simulink model "test_libMdl_TrainEndDataGenerator"  (R2018a)
settings: Solver=FixedStepDiscrete  StartTime=0  StopTime=t_end  FixedStep=0.1  RelTol=1e-3
PreLoadFcn:
  | init_test_libMdl_TrainEndDataGenerator
InitFcn:
  | init_test_libMdl_TrainEndDataGenerator
values from neighbouring files (symbols this model uses):
  a_train_front = [0;0;0]    [init_test_libMdl_TrainEndDataGenerator.m]
  front_track_id = 1    [init_test_libMdl_TrainEndDataGenerator.m]
  v_train_front = 36    [init_test_libMdl_TrainEndDataGenerator.m]
libraries: simulink x1, libMdl_TrainEndDataGenerator x1
settings Model: SimulationMode=accelerator  PauseTimes=224  Creator=hwinter  LastModifiedBy=Hanno
settings DataIOCC: SaveOutput=off  SignalLogging=off  DSMLogging=off  SaveTime=off
settings DebuggingCC: ReadBeforeWriteMsg=DisableAll  WriteAfterWriteMsg=DisableAll  WriteAfterReadMsg=DisableAll  MultiTaskDSMMsg=none
settings HardwareCC: ProdBitPerLong=64  ProdHWDeviceType=Intel->x86-64 (Linux 64)  TargetBitPerPointer=64  TargetBitPerSizeT=64  TargetBitPerPtrDiffT=64  TargetLongLongMode=on  TargetIntDivRoundTo=Zero  TargetEndianess=LittleEndian  TargetWordSize=64  TargetHWDeviceType=MATLAB Host  ProdEqTarget=off
settings SFSimCC: SFSimEcho=off
settings RTWCC: SystemTargetFile=rsim.tlc  TemplateMakefile=rsim_default_tmf  Description=Rapid Simulation Target
settings CodeAppCC: StateflowObjectComments=on
settings RSimTargetCC: TargetLangStandard=C99 (ISO)  GeneratePreprocessorConditionals=Use local settings

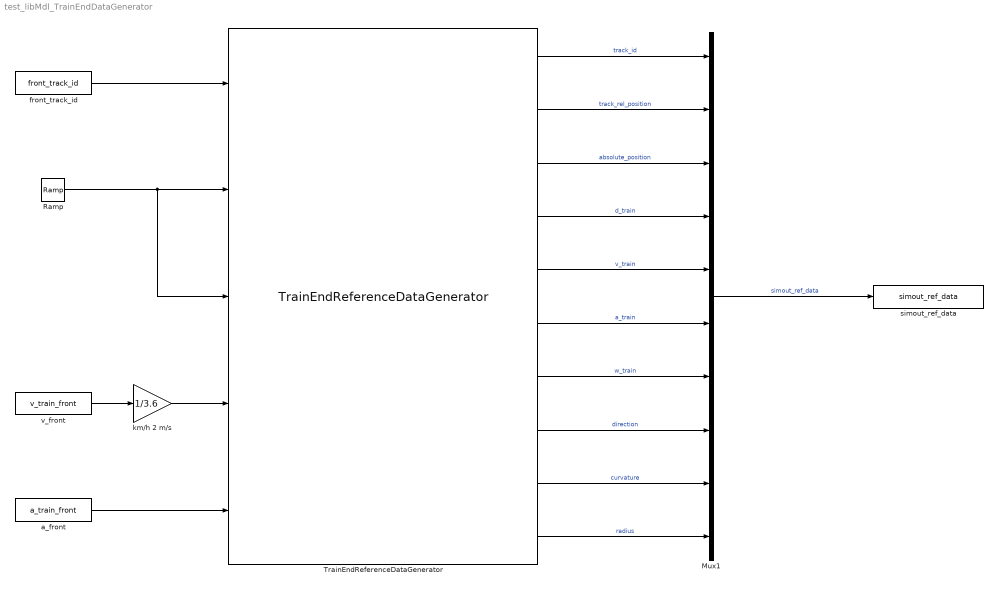
== system test_libMdl_TrainEndDataGenerator ==
  Mux1 : Mux  Inputs=10
  Ramp : simulink/Sources/Ramp  slope=v_train_front/3.6  start=0  InitialOutput=0
  TrainEndReferenceDataGenerator : libMdl_TrainEndDataGenerator/TrainEndReferenceDataGenerator  mv_train_length=train_length  mv_track_map=mat_track_map  mv_track_map_rot_angle=phi_track
  a_front : Constant  Value=a_train_front
  front_track_id : Constant  Value=front_track_id
  km/h 2 m/s : Gain  Gain=1/3.6
  simout_ref_data : ToWorkspace  VariableName=simout_ref_data  SaveFormat=Timeseries  SampleTime=-1
  v_front : Constant  Value=v_train_front
  wires:
  v_front/1 -> km/h 2 m/s/1
  TrainEndReferenceDataGenerator/6 -> Mux1/6  "a_train"
  TrainEndReferenceDataGenerator/7 -> Mux1/7  "w_train"
  TrainEndReferenceDataGenerator/3 -> Mux1/3  "absolute_position"
  TrainEndReferenceDataGenerator/10 -> Mux1/10  "radius"
  TrainEndReferenceDataGenerator/9 -> Mux1/9  "curvature"
  TrainEndReferenceDataGenerator/8 -> Mux1/8  "direction"
  TrainEndReferenceDataGenerator/5 -> Mux1/5  "v_train"
  TrainEndReferenceDataGenerator/4 -> Mux1/4  "d_train"
  TrainEndReferenceDataGenerator/2 -> Mux1/2  "track_rel_position"
  TrainEndReferenceDataGenerator/1 -> Mux1/1  "track_id"
  Mux1/1 -> simout_ref_data/1  "simout_ref_data"
  km/h 2 m/s/1 -> TrainEndReferenceDataGenerator/4
  a_front/1 -> TrainEndReferenceDataGenerator/5
  front_track_id/1 -> TrainEndReferenceDataGenerator/1
  Ramp/1 -> TrainEndReferenceDataGenerator/3, TrainEndReferenceDataGenerator/2
